simulink library "CTRL_LO_ST1_TRQDMDWHL"  (R2023b)
settings: Solver=VariableStepAuto  StartTime=0.0  StopTime=10.0  RelTol=1e-3
undefined symbols (not defined in the file): p_RatGearFr_na, p_RatGearRe_na
settings Model: Creator=blatak  LastModifiedBy=blatak

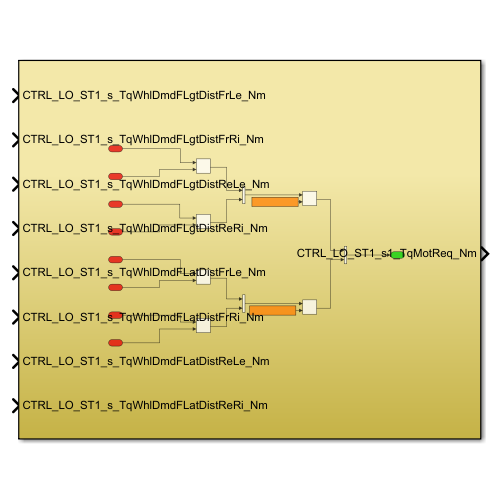
[thumbnail: Simulink's stored preview of the top-level diagram]
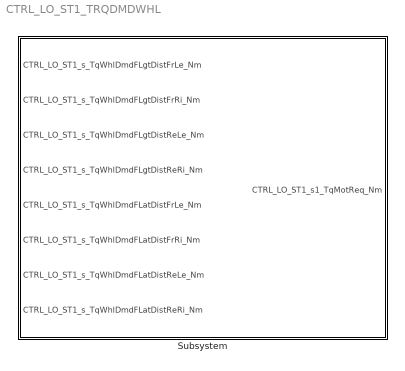
== system CTRL_LO_ST1_TRQDMDWHL ==
  Subsystem : Subsystem

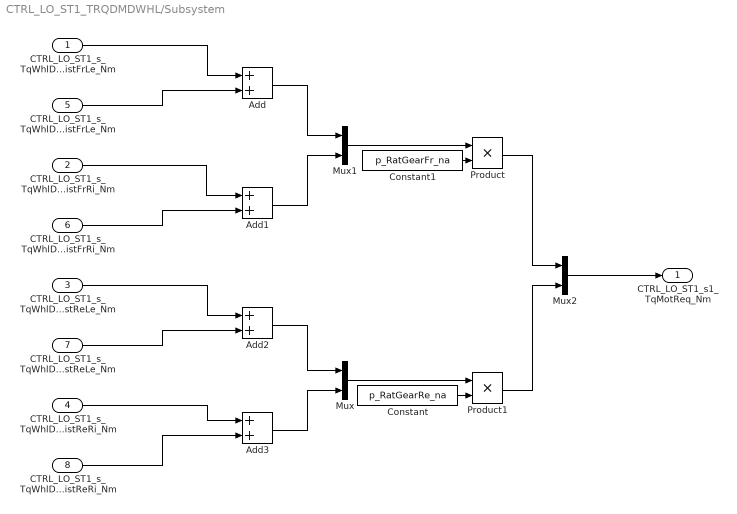
== system CTRL_LO_ST1_TRQDMDWHL/Subsystem ==
  CTRL_LO_ST1_s_TqWhlDmdFLgtDistFrLe_Nm : Inport
  CTRL_LO_ST1_s_TqWhlDmdFLgtDistFrRi_Nm : Inport  Port=2
  CTRL_LO_ST1_s_TqWhlDmdFLgtDistReLe_Nm : Inport  Port=3
  CTRL_LO_ST1_s_TqWhlDmdFLgtDistReRi_Nm : Inport  Port=4
  CTRL_LO_ST1_s_TqWhlDmdFLatDistFrLe_Nm : Inport  Port=5
  CTRL_LO_ST1_s_TqWhlDmdFLatDistFrRi_Nm : Inport  Port=6
  CTRL_LO_ST1_s_TqWhlDmdFLatDistReLe_Nm : Inport  Port=7
  CTRL_LO_ST1_s_TqWhlDmdFLatDistReRi_Nm : Inport  Port=8
  Add{,1..3} (4 alike) : Sum
  Constant : Constant  Value=p_RatGearRe_na
  Constant1 : Constant  Value=p_RatGearFr_na
  Mux : Mux  Inputs=2
  Mux1 : Mux  Inputs=2
  Mux2 : Mux  Inputs=2
  Product : Product
  Product1 : Product
  CTRL_LO_ST1_s1_TqMotReq_Nm : Outport
  wires:
  Mux/1 -> Product1/1
  CTRL_LO_ST1_s_TqWhlDmdFLgtDistFrLe_Nm/1 -> Add/1
  Add/1 -> Mux1/1
  Product1/1 -> Mux2/2
  Product/1 -> Mux2/1
  CTRL_LO_ST1_s_TqWhlDmdFLatDistFrRi_Nm/1 -> Add1/2
  CTRL_LO_ST1_s_TqWhlDmdFLgtDistReRi_Nm/1 -> Add3/1
  Constant1/1 -> Product/2
  CTRL_LO_ST1_s_TqWhlDmdFLgtDistFrRi_Nm/1 -> Add1/1
  Mux2/1 -> CTRL_LO_ST1_s1_TqMotReq_Nm/1
  CTRL_LO_ST1_s_TqWhlDmdFLatDistReRi_Nm/1 -> Add3/2
  Add2/1 -> Mux/1
  Add1/1 -> Mux1/2
  CTRL_LO_ST1_s_TqWhlDmdFLgtDistReLe_Nm/1 -> Add2/1
  CTRL_LO_ST1_s_TqWhlDmdFLatDistFrLe_Nm/1 -> Add/2
  Mux1/1 -> Product/1
  Constant/1 -> Product1/2
  Add3/1 -> Mux/2
  CTRL_LO_ST1_s_TqWhlDmdFLatDistReLe_Nm/1 -> Add2/2
